simulink library "LowFrequencyNoiseEstimatorCoh"  (R2022b)
settings: Solver=VariableStepAuto  StartTime=0.0  StopTime=10.0  RelTol=1e-3
undefined symbols (not defined in the file or in its folder): decRate, magnitude, Row
libraries: TuneVar x22, StateVar x18, TOP x7, TSP x5, FeaturePath x3, HandyTextFile x2, matrix_library x2, PooliirLib x2, SpeedBoundsNoiseSlew x2, RfftLib x1, TunableDelay x1
settings Model: Creator=zs14328  LastModifiedBy=sc48041
settings SolverCC: AlgebraicLoopSolver=TrustRegion
settings DataIOCC: ReturnWorkspaceOutputs=off
settings DebuggingCC: UnconnectedInputMsg=warning  UnconnectedOutputMsg=warning  UnconnectedLineMsg=warning  SFMachineParentedDataDiag=warning  ArithmeticOperatorsInVariantConditions=warning
settings ModelReferenceCC: EnableRefExpFcnMdlSchedulingChecks=on
settings SFSimCC: CustomCodeUndefinedFunction=UseInterfaceOnly

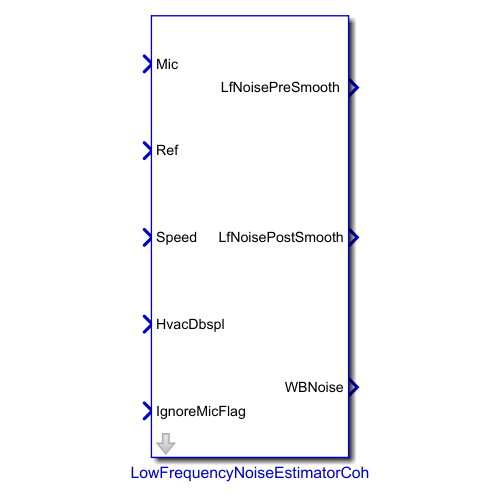
[thumbnail: Simulink's stored preview of the top-level diagram]
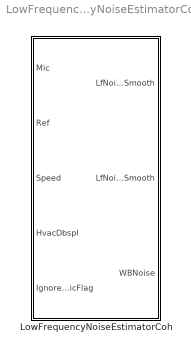
== system LowFrequencyNoiseEstimatorCoh ==
  LowFrequencyNoiseEstimatorCoh : Subsystem  mask(AudioPilot - Low-Frequency Noise Estimator){FeatureName=LfNoise, Config=[], TriggerInit=0}
      mask prompts: FeatureName "Feature Name:"; Config "LowFrequencyNoiseEstimatorCohConfig"
      mask help: This block implements the low-frequency noise estimator using the multi-coherence method.
      mask init:
      | blkh = gcbh;
      | 
      | Config = BTConfig.Assert(blkh,Config);
      | Config.Validate();
      | 
      | DecRate = Config.DecRateHz;
      | DecRate2 = Config.CoherenceDecRateHz;
      | DecRate3 = Config.CoherenceDecRate2Hz;
      | 
      | LowFrequencyNoiseEstimatorCohMask.ConfigureModel ...
      |                 (blkh,Config)
      | 
      | BTConfig.InitSetFeatureIfPresent(blkh,'FeatureName');
      mask Help:
      | This block implements the low-frequency noise estimator using the multi-coherence method.
      | 
      | Arguments for this block:
      | 
      | Design Time Configuration
      | The Feature Name can be specified unless a BTC instance is used, in which case, the instance name will be used as Feature Name.
      | 
      | Build Time Configuration
      | The block can be configured using a BTC object, LowFrequencyNoiseEstimatorCohConfig.
      mask TypeOptions FeatureName: FeaturePath/FeatureName
      mask Callback Config: BTConfig.CallbackHideIfPresent(gcbh,{'FeatureName'});
      mask Callback TriggerInit: LowFrequencyNoiseEstimatorCohMask.TriggerInitCallBack(gcbh);
      mask DialogControl DTCTitle Prompt: <b> Design Time Configuration </b>
      mask DialogControl BTCTitle Prompt: <b> Build Time Configuration </b>
      mask DialogControl Config Tooltip: The configuration has to be an object of the class, LowFrequencyNoiseEstimatorCohConfig.

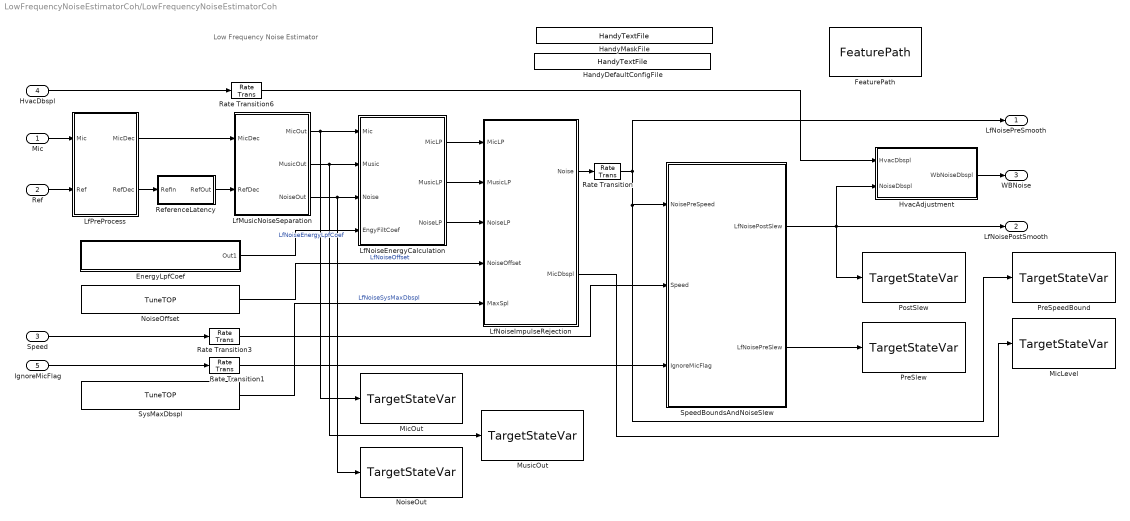
== system LowFrequencyNoiseEstimatorCoh/LowFrequencyNoiseEstimatorCoh ==
  note: Low Frequency Noise Estimator
  Mic : Inport
  Ref : Inport  Port=2
  Speed : Inport  Port=3
  HvacDbspl : Inport  Port=4
  IgnoreMicFlag : Inport  Port=5
  EnergyLpfCoef : Subsystem
  FeaturePath : FeaturePath/FeaturePath  FeatureName=LfNoise  IsGroup=off  GroupNumber=-1  IsModule=off  TriggerInit=[975 -106 1100 -39]
      settings: SourceProductName=Bose Talaria
  HandyDefaultConfigFile : HandyTextFile/HandyTextFile  TemplateSource=Config  FileSuffix=Init  OpenDialogOnLoad=off  UseThisBlockName=off  AddGrandParentNamePrefix=off  TheDefaultText=|  ShowInLibBrowser=on
      | % $(FILENAME) Setup model parameters for each "Init" callback (e.g. update diagram)
      | sample_rate_in_hertz = 44100;
      | frame_size = 32;
      | sysin_channel_count = 2;
      settings: SourceProductName=Bose Talaria
  HandyMaskFile : HandyTextFile/HandyTextFile  TemplateSource=<dialog fields>  FileSuffix=Mask  OpenDialogOnLoad=off  UseThisBlockName=off  AddGrandParentNamePrefix=off  TheDefaultText=|  ShowInLibBrowser=on
      | % $(FILENAME) Setup model parameters for each "Init" callback (e.g. update diagram)
      | sample_rate_in_hertz = 44100;
      | frame_size = 32;
      | sysin_channel_count = 2;
      settings: SourceProductName=Bose Talaria
  HvacAdjustment : Subsystem
  LfMusicNoiseSeparation : Subsystem
  LfNoiseEnergyCalculation : MATLAB Function  TreatAsAtomicUnit=on
  LfNoiseImpulseRejection : Subsystem
  LfPreProcess : Subsystem
  MicLevel : StateVar/TargetStateVar  TriggerInit=[1225 291 1365 359]  TspName=MicLevel  StateName=MicLevel  UseSameName=on  IfdefMacro=[]
      settings: SourceProductName=Bose Talaria
  MicOut : StateVar/TargetStateVar  TriggerInit=[335 366 475 434]  TspName=MicOut  StateName=MicOut  UseSameName=on  IfdefMacro=[]
      settings: SourceProductName=Bose Talaria
  MusicOut : StateVar/TargetStateVar  TriggerInit=[500 416 640 484]  TspName=MusicOut  StateName=MusicOut  UseSameName=on  IfdefMacro=[]
      settings: SourceProductName=Bose Talaria
  NoiseOffset : TuneVar/TuneTOP  TriggerInit=[-45 246 170 284]  TopName=OffsetDb  TuneName=OffsetDb  DataTypeOut=single  TunabilityNumber=1  MinValue=[]  MaxValue=[]  BankNumber=0  PreOverlay=false  PostOverlay=false  UseSameName=on  MaskValue=Config.NoiseOffsetDbspl
      settings: SourceProductName=Bose Talaria
  NoiseOut : StateVar/TargetStateVar  TriggerInit=[335 466 475 534]  TspName=NoiseOut  StateName=NoiseOut  UseSameName=on  IfdefMacro=[]
      settings: SourceProductName=Bose Talaria
  PostSlew : StateVar/TargetStateVar  TriggerInit=[1020 201 1160 269]  TspName=PostSlew  StateName=PostSlew  UseSameName=on  IfdefMacro=[]
      settings: SourceProductName=Bose Talaria
  PreSlew : StateVar/TargetStateVar  TriggerInit=[1020 296 1160 364]  TspName=PreSlew  StateName=PreSlew  UseSameName=on  IfdefMacro=[]
      settings: SourceProductName=Bose Talaria
  PreSpeedBound : StateVar/TargetStateVar  TriggerInit=[1225 201 1365 269]  TspName=PreSpeedBound  StateName=PreSpeedBound  UseSameName=on  IfdefMacro=[]
      settings: SourceProductName=Bose Talaria
  Rate Transition : RateTransition  OutPortSampleTime=1/DecRate2
  Rate Transition1 : RateTransition  Deterministic=off  OutPortSampleTime=1/DecRate2
  Rate Transition3 : RateTransition  Deterministic=off  OutPortSampleTime=1/DecRate2
  Rate Transition6 : RateTransition  Deterministic=off  OutPortSampleTimeOpt=Inherit  OutPortSampleTime=1/decRate
  ReferenceLatency : Subsystem
  SpeedBoundsAndNoiseSlew : Subsystem
  SysMaxDbspl : TuneVar/TuneTOP  TriggerInit=[-45 376 170 414]  TopName=SysMaxDbspl  TuneName=SysMaxDbspl  DataTypeOut=single  TunabilityNumber=1  MinValue=[]  MaxValue=[]  BankNumber=0  PreOverlay=false  PostOverlay=false  UseSameName=on  MaskValue=Config.SysMaxDbspl
      settings: SourceProductName=Bose Talaria
  "LfNoisePreSmooth " : Outport  VectorParamsAs1DForOutWhenUnconnected=off
  LfNoisePostSmooth : Outport  Port=2  VectorParamsAs1DForOutWhenUnconnected=off
  WBNoise : Outport  Port=3  VectorParamsAs1DForOutWhenUnconnected=off
  wires:
  Mic/1 -> LfPreProcess/1(Mic)
  Speed/1 -> Rate Transition3/1
  Ref/1 -> LfPreProcess/2(Ref)
  HvacAdjustment/1(WbNoiseDbspl) -> WBNoise/1
  HvacDbspl/1 -> Rate Transition6/1
  LfNoiseImpulseRejection/1(Noise) -> Rate Transition/1
  LfMusicNoiseSeparation/3(NoiseOut) -> NoiseOut/1, LfNoiseEnergyCalculation/3(Noise)
  LfMusicNoiseSeparation/1(MicOut) -> MicOut/1, LfNoiseEnergyCalculation/1(Mic)
  LfMusicNoiseSeparation/2(MusicOut) -> MusicOut/1, LfNoiseEnergyCalculation/2(Music)
  SpeedBoundsAndNoiseSlew/1(LfNoisePostSlew) -> PostSlew/1, LfNoisePostSmooth/1, HvacAdjustment/2(NoiseDbspl)
  LfNoiseImpulseRejection/2(MicDbspl) -> MicLevel/1
  SpeedBoundsAndNoiseSlew/2(LfNoisePreSlew) -> PreSlew/1
  EnergyLpfCoef/1(Out1) -> LfNoiseEnergyCalculation/4(EngyFiltCoef)  "LfNoiseEnergyLpfCoef"
  LfNoiseEnergyCalculation/1(MicLP) -> LfNoiseImpulseRejection/1(MicLP)
  LfNoiseEnergyCalculation/2(MusicLP) -> LfNoiseImpulseRejection/2(MusicLP)
  LfNoiseEnergyCalculation/3(NoiseLP) -> LfNoiseImpulseRejection/3(NoiseLP)
  NoiseOffset/1 -> LfNoiseImpulseRejection/4(NoiseOffset)  "LfNoiseOffset"
  LfPreProcess/2(RefDec) -> ReferenceLatency/1(RefIn)
  LfPreProcess/1(MicDec) -> LfMusicNoiseSeparation/1(MicDec)
  ReferenceLatency/1(RefOut) -> LfMusicNoiseSeparation/2(RefDec)
  Rate Transition3/1 -> SpeedBoundsAndNoiseSlew/2(Speed)
  Rate Transition6/1 -> HvacAdjustment/1(HvacDbspl)
  Rate Transition/1 -> "LfNoisePreSmooth "/1, PreSpeedBound/1, SpeedBoundsAndNoiseSlew/1(NoisePreSpeed)
  IgnoreMicFlag/1 -> Rate Transition1/1
  SysMaxDbspl/1 -> LfNoiseImpulseRejection/5(MaxSpl)  "LfNoiseSysMaxDbspl"
  Rate Transition1/1 -> SpeedBoundsAndNoiseSlew/3(IgnoreMicFlag)

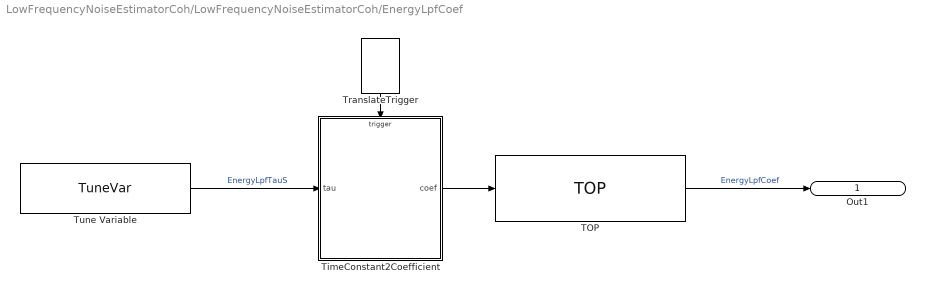
== system LowFrequencyNoiseEstimatorCoh/LowFrequencyNoiseEstimatorCoh/EnergyLpfCoef ==
  TOP : TOP/TOP  TriggerInit=[440 17 630 83]  TopName=EnergyLpfCoef  DataType=single  BankNumber=0  PreOverlay=false  PostOverlay=false  Role=Automatic
      settings: SourceProductName=Bose Talaria
  TimeConstant2Coefficient : MATLAB Function  TreatAsAtomicUnit=on
  TranslateTrigger : TuneVar/TranslateTrigger  TriggerInit=[306 -100 344 -45]
      settings: SourceProductName=Bose Talaria
  Tune Variable : TuneVar/TuneVar  TuneName=EnergyLpfTauS  SpecifyMaxSize=off  VariableDim=1 (Row)  MaxSize=[1 1]  TunabilityNumber=1  MinValue=[]  MaxValue=[]  TriggerInit=[-35 25 135 75]  MaskValue=Config.ImpRejEnergyFilterTauSec
      settings: SourceProductName=Bose Talaria
  Out1 : Outport  VectorParamsAs1DForOutWhenUnconnected=off
  wires:
  TOP/1 -> Out1/1  "EnergyLpfCoef"
  Tune Variable/1 -> TimeConstant2Coefficient/1(tau)  "EnergyLpfTauS"
  TimeConstant2Coefficient/1(coef) -> TOP/1
  TranslateTrigger/1 -> TimeConstant2Coefficient/Trigger

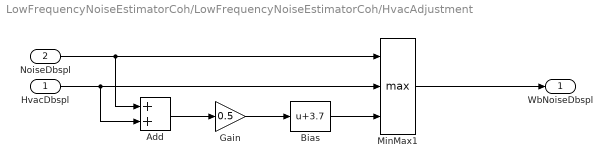
== system LowFrequencyNoiseEstimatorCoh/LowFrequencyNoiseEstimatorCoh/HvacAdjustment ==
  HvacDbspl : Inport
  NoiseDbspl : Inport  Port=2
  Add : Sum
  Bias : Bias  Bias=3.7  SaturateOnIntegerOverflow=off
  Gain : Gain  Gain=0.5
  MinMax1 : MinMax  Function=max  Inputs=3
  WbNoiseDbspl : Outport  VectorParamsAs1DForOutWhenUnconnected=off
  wires:
  NoiseDbspl/1 -> MinMax1/1, Add/1
  HvacDbspl/1 -> MinMax1/2, Add/2
  MinMax1/1 -> WbNoiseDbspl/1
  Add/1 -> Gain/1
  Gain/1 -> Bias/1
  Bias/1 -> MinMax1/3

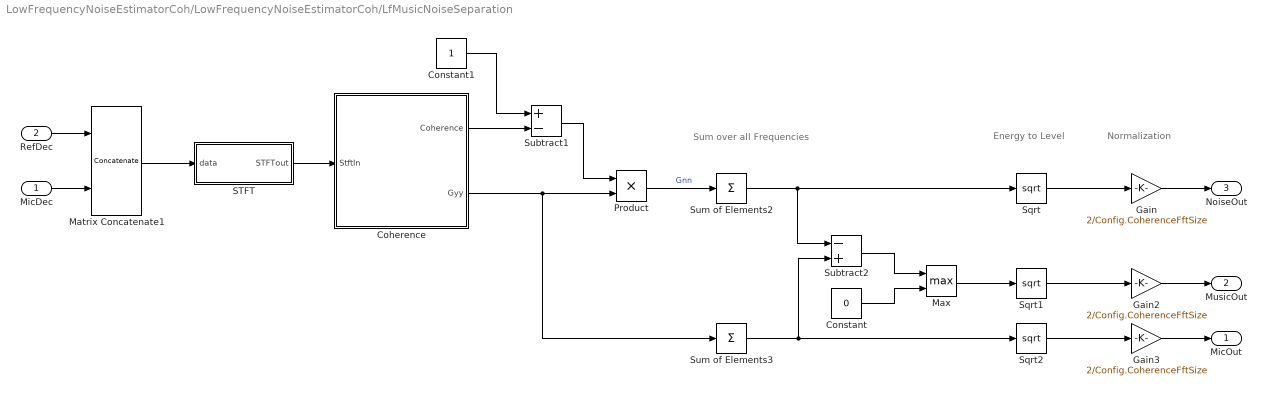
== system LowFrequencyNoiseEstimatorCoh/LowFrequencyNoiseEstimatorCoh/LfMusicNoiseSeparation ==
  note: Energy to
      | Level
  note: Sum over all
      | Frequencies
  note: Normalization
  MicDec : Inport
  RefDec : Inport  Port=2
  Coherence : Subsystem
  Constant : Constant  Value=0  OutDataTypeStr=single
  Constant1 : Constant  OutDataTypeStr=single
  Gain : Gain  Gain=2/Config.CoherenceFftSize
  Gain2 : Gain  Gain=2/Config.CoherenceFftSize
  Gain3 : Gain  Gain=2/Config.CoherenceFftSize
  Matrix Concatenate1 : Concatenate  Mode=Multidimensional array  ConcatenateDimension=2
  Max : MinMax  Function=max  Inputs=2
  Product : Product  RndMeth=Zero
  STFT : Subsystem
  Sqrt : Sqrt
  Sqrt1 : Sqrt
  Sqrt2 : Sqrt
  Subtract1 : Sum  Inputs=+-
  Subtract2 : Sum  Inputs=-+
  Sum of Elements2 : Sum  Inputs=+
  Sum of Elements3 : Sum  Inputs=+
  MicOut : Outport  VectorParamsAs1DForOutWhenUnconnected=off
  MusicOut : Outport  Port=2  VectorParamsAs1DForOutWhenUnconnected=off
  NoiseOut : Outport  Port=3  VectorParamsAs1DForOutWhenUnconnected=off
  wires:
  Coherence/1(Coherence) -> Subtract1/2
  Subtract1/1 -> Product/1
  Product/1 -> Sum of Elements2/1  "Gnn"
  Sum of Elements2/1 -> Subtract2/1, Sqrt/1
  Sqrt/1 -> Gain/1
  RefDec/1 -> Matrix Concatenate1/1
  MicDec/1 -> Matrix Concatenate1/2
  Constant1/1 -> Subtract1/1
  Coherence/2(Gyy) -> Product/2, Sum of Elements3/1
  Sum of Elements3/1 -> Sqrt2/1, Subtract2/2
  Sqrt2/1 -> Gain3/1
  Subtract2/1 -> Max/1
  Sqrt1/1 -> Gain2/1
  Gain/1 -> NoiseOut/1
  Gain2/1 -> MusicOut/1
  Gain3/1 -> MicOut/1
  Matrix Concatenate1/1 -> STFT/1(data)
  STFT/1(STFTout) -> Coherence/1(StftIn)
  Max/1 -> Sqrt1/1
  Constant/1 -> Max/2

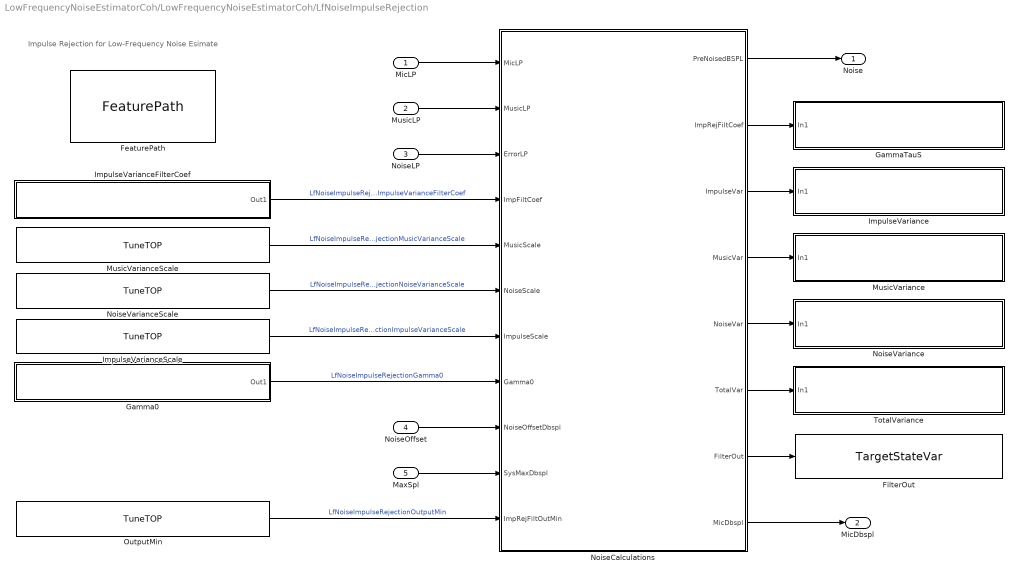
== system LowFrequencyNoiseEstimatorCoh/LowFrequencyNoiseEstimatorCoh/LfNoiseImpulseRejection ==
  note: Impulse Rejection for Low-Frequency Noise Esimate
  MicLP : Inport  SampleTime=1/DecRate3
  MusicLP : Inport  Port=2  SampleTime=1/DecRate3
  NoiseLP : Inport  Port=3  SampleTime=1/DecRate3
  NoiseOffset : Inport  Port=4
  MaxSpl : Inport  Port=5
  FeaturePath : FeaturePath/FeaturePath  FeatureName=ImpulseRejection  IsGroup=off  GroupNumber=-1  IsModule=off  TriggerInit=[-70 349 105 436]
      settings: SourceProductName=Bose Talaria
  FilterOut : StateVar/TargetStateVar  TriggerInit=[805 788 1055 842]  TspName=FilterOut  StateName=FilterOut  UseSameName=on  IfdefMacro=[]
      settings: SourceProductName=Bose Talaria
  Gamma0 : Subsystem
  GammaTauS : Subsystem
  ImpulseVariance : Subsystem
  ImpulseVarianceFilterCoef : Subsystem
  ImpulseVarianceScale : TuneVar/TuneTOP  TriggerInit=[-135 649 170 691]  TopName=ImpulseVarianceScale  TuneName=ImpulseVarianceScale  DataType=single  TunabilityNumber=1  MinValue=[]  MaxValue=[]  BankNumber=0  PreOverlay=false  PostOverlay=false  UseSameName=on  MaskValue=Config.ImpRejImpulseScale
      settings: SourceProductName=Bose Talaria
  MusicVariance : Subsystem
  MusicVarianceScale : TuneVar/TuneTOP  TriggerInit=[-135 539 170 581]  TopName=MusicVarianceScale  TuneName=MusicVarianceScale  DataType=single  TunabilityNumber=1  MinValue=[]  MaxValue=[]  BankNumber=0  PreOverlay=false  PostOverlay=false  UseSameName=on  MaskValue=Config.ImpRejMusicScale
      settings: SourceProductName=Bose Talaria
  NoiseCalculations : MATLAB Function  TreatAsAtomicUnit=on
  NoiseVariance : Subsystem
  NoiseVarianceScale : TuneVar/TuneTOP  TriggerInit=[-135 594 170 636]  TopName=NoiseVarianceScale  TuneName=NoiseVarianceScale  DataType=single  TunabilityNumber=1  MinValue=[]  MaxValue=[]  BankNumber=0  PreOverlay=false  PostOverlay=false  UseSameName=on  MaskValue=Config.ImpRejNoiseScale
      settings: SourceProductName=Bose Talaria
  "OutputMin " : TuneVar/TuneTOP  TriggerInit=[-135 869 170 911]  TopName=OutputMin  TuneName=OutputMin  DataType=single  TunabilityNumber=1  MinValue=[]  MaxValue=[]  BankNumber=0  PreOverlay=false  PostOverlay=false  UseSameName=on  MaskValue=Config.ImpRejOutputMin
      settings: SourceProductName=Bose Talaria
  TotalVariance : Subsystem
  Noise : Outport  VectorParamsAs1DForOutWhenUnconnected=off
  MicDbspl : Outport  Port=2  VectorParamsAs1DForOutWhenUnconnected=off
  wires:
  MicLP/1 -> NoiseCalculations/1(MicLP)
  MusicLP/1 -> NoiseCalculations/2(MusicLP)
  NoiseLP/1 -> NoiseCalculations/3(ErrorLP)
  "OutputMin "/1 -> NoiseCalculations/11(ImpRejFiltOutMin)  "LfNoiseImpulseRejectionOutputMin"
  NoiseCalculations/1(PreNoisedBSPL) -> Noise/1
  NoiseCalculations/8(MicDbspl) -> MicDbspl/1
  NoiseVarianceScale/1 -> NoiseCalculations/6(NoiseScale)  "LfNoiseImpulseRejectionNoiseVarianceScale"
  MusicVarianceScale/1 -> NoiseCalculations/5(MusicScale)  "LfNoiseImpulseRejectionMusicVarianceScale"
  ImpulseVarianceScale/1 -> NoiseCalculations/7(ImpulseScale)  "LfNoiseImpulseRejectionImpulseVarianceScale"
  Gamma0/1(Out1) -> NoiseCalculations/8(Gamma0)  "LfNoiseImpulseRejectionGamma0"
  ImpulseVarianceFilterCoef/1(Out1) -> NoiseCalculations/4(ImpFiltCoef)  "LfNoiseImpulseRejectionImpulseVarianceFilterCoef"
  MaxSpl/1 -> NoiseCalculations/10(SysMaxDbspl)
  NoiseOffset/1 -> NoiseCalculations/9(NoiseOffsetDbspl)
  NoiseCalculations/4(MusicVar) -> MusicVariance/1(In1)
  NoiseCalculations/3(ImpulseVar) -> ImpulseVariance/1(In1)
  NoiseCalculations/5(NoiseVar) -> NoiseVariance/1(In1)
  NoiseCalculations/6(TotalVar) -> TotalVariance/1(In1)
  NoiseCalculations/2(ImpRejFiltCoef) -> GammaTauS/1(In1)
  NoiseCalculations/7(FilterOut) -> FilterOut/1

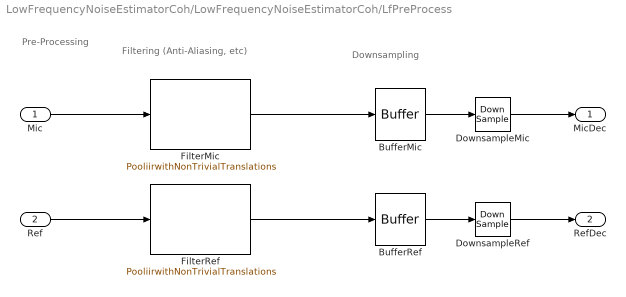
== system LowFrequencyNoiseEstimatorCoh/LowFrequencyNoiseEstimatorCoh/LfPreProcess ==
  note: Filtering
      | (Anti-Aliasing, etc)
  note: Downsampling
  note: Pre-Processing
  Mic : Inport
  Ref : Inport  Port=2
  BufferMic : Buffer  N=Config.DecimationFactor  OutputFrames=off
  BufferRef : Buffer  N=Config.DecimationFactor  OutputFrames=off
  DownsampleMic : DownSample  N=Config.DecimationFactor
  DownsampleRef : DownSample  N=Config.DecimationFactor
  FilterMic : PooliirLib/PooliirwithNonTrivialTranslations  maxNumStages=Config.AntiAliasFilterNumStages  numStages=Config.AntiAliasFilterNumStages  sosCoefficients=Config.AntiAliasFilterSos  alias='LPMicFilt'  variantType=Config.MicFiltVariant  FeatureName=Mic
  FilterRef : PooliirLib/PooliirwithNonTrivialTranslations  maxNumStages=Config.AntiAliasFilterNumStages  numStages=Config.AntiAliasFilterNumStages  sosCoefficients=Config.AntiAliasFilterSos  alias='LFRefFilt'  variantType=Config.RefFiltVariant  FeatureName=Ref
  MicDec : Outport  VectorParamsAs1DForOutWhenUnconnected=off
  RefDec : Outport  Port=2  VectorParamsAs1DForOutWhenUnconnected=off
  wires:
  DownsampleRef/1 -> RefDec/1
  DownsampleMic/1 -> MicDec/1
  BufferMic/1 -> DownsampleMic/1
  Mic/1 -> FilterMic/1
  Ref/1 -> FilterRef/1
  FilterMic/1 -> BufferMic/1
  BufferRef/1 -> DownsampleRef/1
  FilterRef/1 -> BufferRef/1

== system LowFrequencyNoiseEstimatorCoh/LowFrequencyNoiseEstimatorCoh/ReferenceLatency ==
  RefIn : Inport  SampleTime=1/DecRate
  Delay : TunableDelay/Delay  maxDelayTime=int32(floor(Config.RefMaxLatencyMsec/1000*DecRate))  frameSize=1  numChannels=1  bufferAlias=[]  headerFilename=[]
  RefLatencySamples : Subsystem
  RefOut : Outport  VectorParamsAs1DForOutWhenUnconnected=off
  wires:
  Delay/1 -> RefOut/1
  RefIn/1 -> Delay/1
  RefLatencySamples/1(LfNoiseRefLatencySamples) -> Delay/2  "LfNoise_ref_latency_samples"

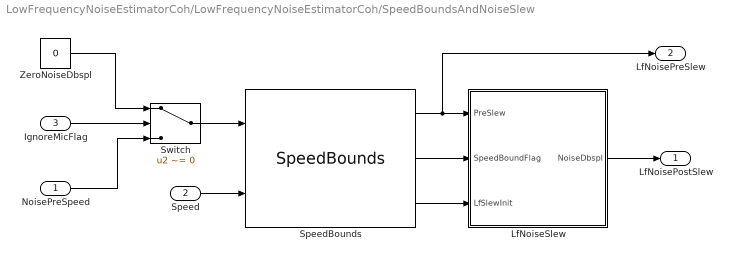
== system LowFrequencyNoiseEstimatorCoh/LowFrequencyNoiseEstimatorCoh/SpeedBoundsAndNoiseSlew ==
  NoisePreSpeed : Inport
  Speed : Inport  Port=2
  IgnoreMicFlag : Inport  Port=3
  LfNoiseSlew : Subsystem
  SpeedBounds : SpeedBoundsNoiseSlew/SpeedBounds  FeatureName=SpeedBounds  Config=Config.SpeedBounds
  Switch : Switch  Criteria=u2 ~= 0  SaturateOnIntegerOverflow=off  InputSameDT=off
  ZeroNoiseDbspl : Constant  Value=0  OutDataTypeStr=single
  LfNoisePostSlew : Outport  VectorParamsAs1DForOutWhenUnconnected=off
  LfNoisePreSlew : Outport  Port=2  VectorParamsAs1DForOutWhenUnconnected=off
  wires:
  Speed/1 -> SpeedBounds/2
  SpeedBounds/2 -> LfNoiseSlew/2(SpeedBoundFlag)
  SpeedBounds/1 -> LfNoisePreSlew/1, LfNoiseSlew/1(PreSlew)
  LfNoiseSlew/1(NoiseDbspl) -> LfNoisePostSlew/1
  NoisePreSpeed/1 -> Switch/3
  Switch/1 -> SpeedBounds/1
  IgnoreMicFlag/1 -> Switch/2
  ZeroNoiseDbspl/1 -> Switch/1
  SpeedBounds/3 -> LfNoiseSlew/3(LfSlewInit)

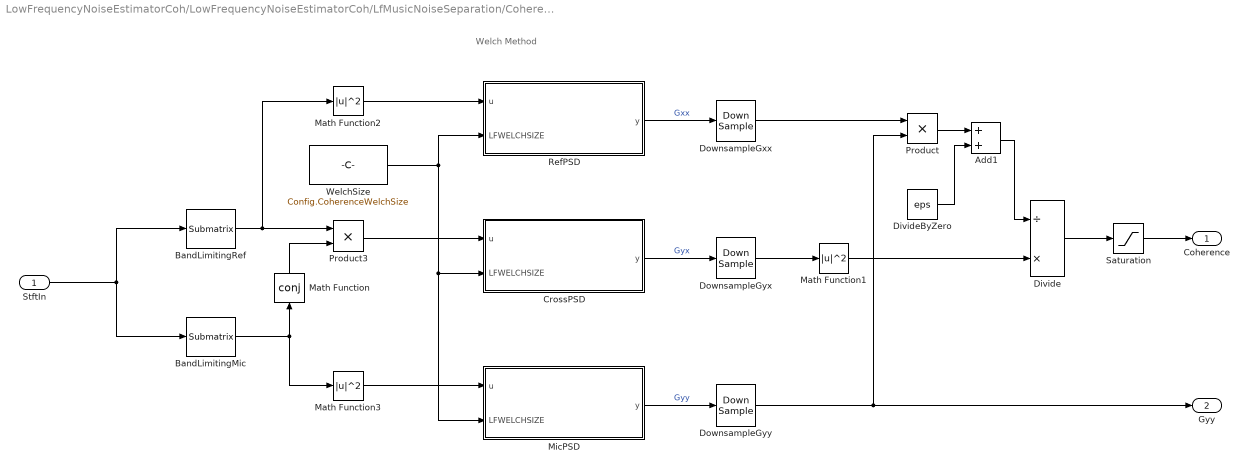
== system LowFrequencyNoiseEstimatorCoh/LowFrequencyNoiseEstimatorCoh/LfMusicNoiseSeparation/Coherence ==
  note: Welch Method
  StftIn : Inport
  Add1 : Sum
  BandLimitingMic : matrix_library/Submatrix  RowSpan=Range of rows  RowStartMode=Index  RowStartIndex=Config.CoherenceLowFrequencyIndex  RowEndMode=Index  RowEndIndex=Config.CoherenceHighFrequencyIndex  ColSpan=One column  ColStartMode=Last  ColStartIndex=1  ColEndMode=Last  ColEndIndex=1
  BandLimitingRef : matrix_library/Submatrix  RowSpan=Range of rows  RowStartMode=Index  RowStartIndex=Config.CoherenceLowFrequencyIndex  RowEndMode=Index  RowEndIndex=Config.CoherenceHighFrequencyIndex  ColSpan=One column  ColStartMode=First  ColStartIndex=1  ColEndMode=Index  ColEndIndex=1
  CrossPSD : MATLAB Function  TreatAsAtomicUnit=on
  Divide : Product  Inputs=/*
  DivideByZero : Constant  Value=eps  OutDataTypeStr=single
  DownsampleGxx : DownSample  N=Config.CoherenceWelchSize  RateOptions=Allow multirate processing
  DownsampleGyx : DownSample  N=Config.CoherenceWelchSize  RateOptions=Allow multirate processing
  DownsampleGyy : DownSample  N=Config.CoherenceWelchSize  RateOptions=Allow multirate processing
  Math Function : Math  Operator=conj  SignedPower=on
  Math Function1 : Math  Operator=magnitude^2  SignedPower=on
  Math Function2 : Math  Operator=magnitude^2  SignedPower=on
  Math Function3 : Math  Operator=magnitude^2  SignedPower=on
  MicPSD : MATLAB Function  TreatAsAtomicUnit=on
  Product : Product  RndMeth=Zero
  Product3 : Product  RndMeth=Zero
  "RefPSD " : MATLAB Function  TreatAsAtomicUnit=on
  Saturation : Saturate  UpperLimit=1  LowerLimit=0
  WelchSize : Constant  Value=Config.CoherenceWelchSize  OutDataTypeStr=single
  Coherence : Outport  VectorParamsAs1DForOutWhenUnconnected=off
  Gyy : Outport  Port=2  VectorParamsAs1DForOutWhenUnconnected=off
  wires:
  Math Function/1 -> Product3/2
  Divide/1 -> Saturation/1
  Product3/1 -> CrossPSD/1(u)
  StftIn/1 -> BandLimitingMic/1, BandLimitingRef/1
  Product/1 -> Add1/1
  Math Function1/1 -> Divide/2
  CrossPSD/1(y) -> DownsampleGyx/1  "Gyx"
  "RefPSD "/1(y) -> DownsampleGxx/1  "Gxx"
  MicPSD/1(y) -> DownsampleGyy/1  "Gyy"
  DivideByZero/1 -> Add1/2
  Add1/1 -> Divide/1
  Math Function2/1 -> "RefPSD "/1(u)
  Math Function3/1 -> MicPSD/1(u)
  BandLimitingRef/1 -> Product3/1, Math Function2/1
  BandLimitingMic/1 -> Math Function/1, Math Function3/1
  WelchSize/1 -> "RefPSD "/2(LFWELCHSIZE), MicPSD/2(LFWELCHSIZE), CrossPSD/2(LFWELCHSIZE)
  DownsampleGxx/1 -> Product/1
  DownsampleGyx/1 -> Math Function1/1
  DownsampleGyy/1 -> Product/2, Gyy/1
  Saturation/1 -> Coherence/1

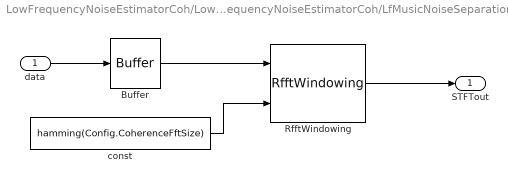
== system LowFrequencyNoiseEstimatorCoh/LowFrequencyNoiseEstimatorCoh/LfMusicNoiseSeparation/STFT ==
  data : Inport
  Buffer : Buffer  N=Config.CoherenceFftSize  V=Config.CoherenceOverlap
  RfftWindowing : RfftLib/RfftWindowing  Description=This block computes the Fourier Transform using an optimized FFT for real 2-channel input.  Config=Config.RfftWindowingStft
      settings: SourceProductName=Bose Blocklib
  const : Constant  Value=hamming(Config.CoherenceFftSize)  OutDataTypeStr=single
  STFTout : Outport  VectorParamsAs1DForOutWhenUnconnected=off
  wires:
  Buffer/1 -> RfftWindowing/1
  const/1 -> RfftWindowing/2
  data/1 -> Buffer/1
  RfftWindowing/1 -> STFTout/1

== system LowFrequencyNoiseEstimatorCoh/LowFrequencyNoiseEstimatorCoh/LfNoiseImpulseRejection/Gamma0 ==
  TOP : TOP/TOP  TriggerInit=[475 20 675 70]  TopName=Gamma0  DataType=single  BankNumber=0  PreOverlay=false  PostOverlay=false  Role=Automatic
      settings: SourceProductName=Bose Talaria
  TimeConstant2Coefficient : MATLAB Function  TreatAsAtomicUnit=on
  TranslateTrigger : TuneVar/TranslateTrigger  TriggerInit=[306 -100 344 -45]
      settings: SourceProductName=Bose Talaria
  Tune Variable : TuneVar/TuneVar  TuneName=Gamma0TauS  SpecifyMaxSize=off  VariableDim=1 (Row)  MaxSize=[1 1]  TunabilityNumber=1  MinValue=[]  MaxValue=[]  TriggerInit=[-160 22 155 68]  MaskValue=Config.ImpRejGamma0TauSec
      settings: SourceProductName=Bose Talaria
  Out1 : Outport  VectorParamsAs1DForOutWhenUnconnected=off
  wires:
  TOP/1 -> Out1/1  "Gamma0"
  Tune Variable/1 -> TimeConstant2Coefficient/1(tau)  "Gamma0TauS"
  TimeConstant2Coefficient/1(coef) -> TOP/1
  TranslateTrigger/1 -> TimeConstant2Coefficient/Trigger

== system LowFrequencyNoiseEstimatorCoh/LowFrequencyNoiseEstimatorCoh/LfNoiseImpulseRejection/GammaTauS ==
  In1 : Inport
  GammaConversion : MATLAB Function  TreatAsAtomicUnit=on
  InterpretTrigger : StateVar/InterpretTrigger  TriggerInit=[336 20 374 75]
      settings: SourceProductName=Bose Talaria
  StateVar : StateVar/StateVar  TriggerInit=[495 139 735 201]  StateName=GammaTauS
      settings: SourceProductName=Bose Talaria
  TSP : TSP/TSP  TriggerInit=[0 138 260 202]  TspName=FiltCoef  IfDefMacro=[]  Role=Automatic
      settings: SourceProductName=Bose Talaria
  wires:
  InterpretTrigger/1 -> GammaConversion/Trigger
  TSP/1 -> GammaConversion/1(Coef)
  GammaConversion/1(State) -> StateVar/1
  In1/1 -> TSP/1

== system LowFrequencyNoiseEstimatorCoh/LowFrequencyNoiseEstimatorCoh/LfNoiseImpulseRejection/ImpulseVariance ==
  In1 : Inport
  InterpretTrigger : StateVar/InterpretTrigger  TriggerInit=[336 20 374 75]
      settings: SourceProductName=Bose Talaria
  StateVar : StateVar/StateVar  TriggerInit=[495 139 735 201]  StateName=ImpulseVarianceDb
      settings: SourceProductName=Bose Talaria
  TSP : TSP/TSP  TriggerInit=[0 138 215 202]  TspName=ImpulseVariance  IfDefMacro=[]  Role=Automatic
      settings: SourceProductName=Bose Talaria
  db20 : MATLAB Function  TreatAsAtomicUnit=on
  wires:
  In1/1 -> TSP/1
  db20/1(State) -> StateVar/1
  TSP/1 -> db20/1(TSP1)
  InterpretTrigger/1 -> db20/Trigger

== system LowFrequencyNoiseEstimatorCoh/LowFrequencyNoiseEstimatorCoh/LfNoiseImpulseRejection/ImpulseVarianceFilterCoef ==
  TOP : TOP/TOP  TriggerInit=[440 17 725 83]  TopName=ImpulseVarianceFilterCoef  DataType=single  BankNumber=0  PreOverlay=false  PostOverlay=false  Role=Automatic
      settings: SourceProductName=Bose Talaria
  TimeConstant2Coefficient : MATLAB Function  TreatAsAtomicUnit=on
  TranslateTrigger : TuneVar/TranslateTrigger  TriggerInit=[306 -100 344 -45]
      settings: SourceProductName=Bose Talaria
  Tune Variable : TuneVar/TuneVar  TuneName=ImpulseVarianceFiltTauS  SpecifyMaxSize=off  VariableDim=1 (Row)  MaxSize=[1 1]  TunabilityNumber=1  MinValue=[]  MaxValue=[]  TriggerInit=[-265 20 100 80]  MaskValue=Config.ImpRejImpulseVarianceFilterTauSec
      settings: SourceProductName=Bose Talaria
  Out1 : Outport  VectorParamsAs1DForOutWhenUnconnected=off
  wires:
  TOP/1 -> Out1/1  "ImpulseVarianceFilterCoef"
  Tune Variable/1 -> TimeConstant2Coefficient/1(tau)  "ImpulseVarianceFiltTauS"
  TimeConstant2Coefficient/1(coef) -> TOP/1
  TranslateTrigger/1 -> TimeConstant2Coefficient/Trigger

== system LowFrequencyNoiseEstimatorCoh/LowFrequencyNoiseEstimatorCoh/LfNoiseImpulseRejection/MusicVariance ==
  In1 : Inport
  InterpretTrigger : StateVar/InterpretTrigger  TriggerInit=[336 20 374 75]
      settings: SourceProductName=Bose Talaria
  StateVar : StateVar/StateVar  TriggerInit=[455 136 685 204]  StateName=MusicVarianceDb
      settings: SourceProductName=Bose Talaria
  TSP : TSP/TSP  TriggerInit=[20 136 260 204]  TspName=MusicVariance  IfDefMacro=[]  Role=Automatic
      settings: SourceProductName=Bose Talaria
  "db20 " : MATLAB Function  TreatAsAtomicUnit=on
  wires:
  In1/1 -> TSP/1
  "db20 "/1(State) -> StateVar/1
  TSP/1 -> "db20 "/1(TSP1)
  InterpretTrigger/1 -> "db20 "/Trigger

== system LowFrequencyNoiseEstimatorCoh/LowFrequencyNoiseEstimatorCoh/LfNoiseImpulseRejection/NoiseVariance ==
  In1 : Inport
  InterpretTrigger : StateVar/InterpretTrigger  TriggerInit=[336 20 374 75]
      settings: SourceProductName=Bose Talaria
  StateVar : StateVar/StateVar  TriggerInit=[455 136 685 204]  StateName=NoiseVarianceDb
      settings: SourceProductName=Bose Talaria
  TSP : TSP/TSP  TriggerInit=[20 136 260 204]  TspName=NoiseVariance  IfDefMacro=[]  Role=Automatic
      settings: SourceProductName=Bose Talaria
  "db20 " : MATLAB Function  TreatAsAtomicUnit=on
  wires:
  InterpretTrigger/1 -> "db20 "/Trigger
  TSP/1 -> "db20 "/1(TSP1)
  "db20 "/1(State) -> StateVar/1
  In1/1 -> TSP/1

== system LowFrequencyNoiseEstimatorCoh/LowFrequencyNoiseEstimatorCoh/LfNoiseImpulseRejection/TotalVariance ==
  In1 : Inport
  InterpretTrigger : StateVar/InterpretTrigger  TriggerInit=[336 20 374 75]
      settings: SourceProductName=Bose Talaria
  StateVar : StateVar/StateVar  TriggerInit=[455 136 685 204]  StateName=TotalVarianceDb
      settings: SourceProductName=Bose Talaria
  TSP : TSP/TSP  TriggerInit=[20 136 260 204]  TspName=TotalVariance  IfDefMacro=[]  Role=Automatic
      settings: SourceProductName=Bose Talaria
  "db20 " : MATLAB Function  TreatAsAtomicUnit=on
  wires:
  InterpretTrigger/1 -> "db20 "/Trigger
  TSP/1 -> "db20 "/1(TSP1)
  "db20 "/1(State) -> StateVar/1
  In1/1 -> TSP/1

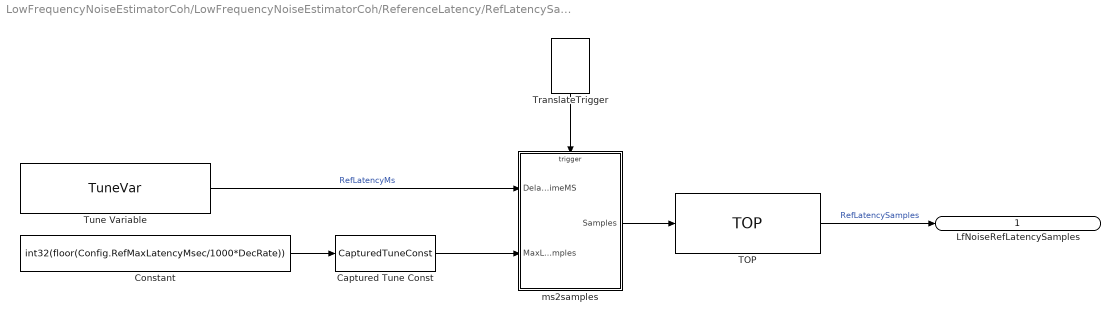
== system LowFrequencyNoiseEstimatorCoh/LowFrequencyNoiseEstimatorCoh/ReferenceLatency/RefLatencySamples ==
  Captured Tune Const : TuneVar/CapturedTuneConst  TriggerInit=[70 162 170 198]  Role=Automatic
      settings: SourceProductName=Bose Talaria
  Constant : Constant  Value=int32(floor(Config.RefMaxLatencyMsec/1000*DecRate))  OutDataTypeStr=int32
  TOP : TOP/TOP  TriggerInit=[410 120 555 180]  TopName=RefLatencySamples  DataType=int32  BankNumber=0  PreOverlay=false  PostOverlay=false  Role=Automatic
      settings: SourceProductName=Bose Talaria
  TranslateTrigger : TuneVar/TranslateTrigger  TriggerInit=[286 -35 324 20]
      settings: SourceProductName=Bose Talaria
  Tune Variable : TuneVar/TuneVar  TuneName=RefLatencyMs  SpecifyMaxSize=off  VariableDim=1 (Row)  MaxSize=[1 1]  TunabilityNumber=1  MinValue=[]  MaxValue=[]  TriggerInit=[-245 90 -55 140]  MaskValue=Config.RefLatencyMsec
      settings: SourceProductName=Bose Talaria
  ms2samples : MATLAB Function  TreatAsAtomicUnit=on
  LfNoiseRefLatencySamples : Outport  VectorParamsAs1DForOutWhenUnconnected=off
  wires:
  Tune Variable/1 -> ms2samples/1(DelayTimeMS)  "RefLatencyMs"
  ms2samples/1(Samples) -> TOP/1
  TranslateTrigger/1 -> ms2samples/Trigger
  TOP/1 -> LfNoiseRefLatencySamples/1  "RefLatencySamples"
  Captured Tune Const/1 -> ms2samples/2(MaxLatencySamples)
  Constant/1 -> Captured Tune Const/1

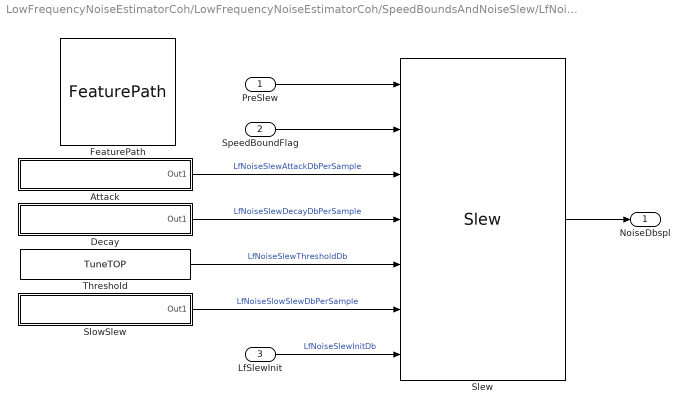
== system LowFrequencyNoiseEstimatorCoh/LowFrequencyNoiseEstimatorCoh/SpeedBoundsAndNoiseSlew/LfNoiseSlew ==
  PreSlew : Inport
  SpeedBoundFlag : Inport  Port=2
  LfSlewInit : Inport  Port=3
  Attack : Subsystem
  Decay : Subsystem
  FeaturePath : FeaturePath/FeaturePath  FeatureName=Slew  IsGroup=off  GroupNumber=-1  IsModule=off  TriggerInit=[-225 44 -110 151]
      settings: SourceProductName=Bose Talaria
  Slew : SpeedBoundsNoiseSlew/Slew  SystemSampleTime=-1  VariantActivationTime=update diagram  Latency=0  AutoFrameSizeCalculation=off
  SlowSlew : Subsystem
  Threshold : TuneVar/TuneTOP  TriggerInit=[-265 255 -95 285]  TopName=ThresholdDb  TuneName=ThresholdDb  DataType=single  TunabilityNumber=1  MinValue=[]  MaxValue=[]  BankNumber=0  PreOverlay=false  PostOverlay=false  UseSameName=on  MaskValue=Config.SlewThresholdDb
      settings: SourceProductName=Bose Talaria
  NoiseDbspl : Outport  VectorParamsAs1DForOutWhenUnconnected=off
  wires:
  Slew/1 -> NoiseDbspl/1
  SpeedBoundFlag/1 -> Slew/2
  PreSlew/1 -> Slew/1
  SlowSlew/1(Out1) -> Slew/6  "LfNoiseSlowSlewDbPerSample"
  Attack/1(Out1) -> Slew/3  "LfNoiseSlewAttackDbPerSample"
  Threshold/1 -> Slew/5  "LfNoiseSlewThresholdDb"
  Decay/1(Out1) -> Slew/4  "LfNoiseSlewDecayDbPerSample"
  LfSlewInit/1 -> Slew/7  "LfNoiseSlewInitDb"

== system LowFrequencyNoiseEstimatorCoh/LowFrequencyNoiseEstimatorCoh/SpeedBoundsAndNoiseSlew/LfNoiseSlew/Attack ==
  TOP : TOP/TOP  TriggerInit=[125 85 330 145]  TopName=AttackDbPerSample  DataType=single  BankNumber=0  PreOverlay=false  PostOverlay=false  Role=Automatic
      settings: SourceProductName=Bose Talaria
  TranslateTrigger : TuneVar/TranslateTrigger  TriggerInit=[-19 -10 19 45]
      settings: SourceProductName=Bose Talaria
  Tune Variable : TuneVar/TuneVar  TuneName=AttackDbPerS  SpecifyMaxSize=off  VariableDim=1 (Row)  MaxSize=[1 1]  TunabilityNumber=1  MinValue=[]  MaxValue=[]  TriggerInit=[-385 90 -215 140]  MaskValue=Config.SlewAttackDbpersec
      settings: SourceProductName=Bose Talaria
  sec2sample : MATLAB Function  TreatAsAtomicUnit=on
  Out1 : Outport  VectorParamsAs1DForOutWhenUnconnected=off
  wires:
  TOP/1 -> Out1/1  "AttackDbPerSample"
  sec2sample/1(y) -> TOP/1
  Tune Variable/1 -> sec2sample/1(u)  "AttackDbPerS"
  TranslateTrigger/1 -> sec2sample/Trigger

== system LowFrequencyNoiseEstimatorCoh/LowFrequencyNoiseEstimatorCoh/SpeedBoundsAndNoiseSlew/LfNoiseSlew/Decay ==
  TOP : TOP/TOP  TriggerInit=[100 85 315 145]  TopName=DecayDbPerSample  DataType=single  BankNumber=0  PreOverlay=false  PostOverlay=false  Role=Automatic
      settings: SourceProductName=Bose Talaria
  TranslateTrigger : TuneVar/TranslateTrigger  TriggerInit=[-19 -10 19 45]
      settings: SourceProductName=Bose Talaria
  Tune Variable : TuneVar/TuneVar  TuneName=DecayDbPerS  SpecifyMaxSize=off  VariableDim=1 (Row)  MaxSize=[1 1]  TunabilityNumber=1  MinValue=[]  MaxValue=[]  TriggerInit=[-385 90 -215 140]  MaskValue=Config.SlewDecayDbpersec
      settings: SourceProductName=Bose Talaria
  sec2sample : MATLAB Function  TreatAsAtomicUnit=on
  Out1 : Outport  VectorParamsAs1DForOutWhenUnconnected=off
  wires:
  TranslateTrigger/1 -> sec2sample/Trigger
  Tune Variable/1 -> sec2sample/1(u)  "DecayDbPerS"
  sec2sample/1(y) -> TOP/1
  TOP/1 -> Out1/1  "DecayDbPerSample"

== system LowFrequencyNoiseEstimatorCoh/LowFrequencyNoiseEstimatorCoh/SpeedBoundsAndNoiseSlew/LfNoiseSlew/SlowSlew ==
  TOP : TOP/TOP  TriggerInit=[100 87 320 143]  TopName=SlowDbPerSample  DataType=single  BankNumber=0  PreOverlay=false  PostOverlay=false  Role=Automatic
      settings: SourceProductName=Bose Talaria
  TranslateTrigger : TuneVar/TranslateTrigger  TriggerInit=[-19 -10 19 45]
      settings: SourceProductName=Bose Talaria
  Tune Variable : TuneVar/TuneVar  TuneName=SlowDbPerS  SpecifyMaxSize=off  VariableDim=1 (Row)  MaxSize=[1 1]  TunabilityNumber=1  MinValue=[]  MaxValue=[]  TriggerInit=[-335 90 -165 140]  MaskValue=Config.SlewSlowSlewDbpersec
      settings: SourceProductName=Bose Talaria
  sec2sample : MATLAB Function  TreatAsAtomicUnit=on
  Out1 : Outport  VectorParamsAs1DForOutWhenUnconnected=off
  wires:
  TOP/1 -> Out1/1  "SlowDbPerSample"
  sec2sample/1(y) -> TOP/1
  Tune Variable/1 -> sec2sample/1(u)  "SlowDbPerS"
  TranslateTrigger/1 -> sec2sample/Trigger

== matlab function LowFrequencyNoiseEstimatorCoh/LfNoiseImpulseRejection/MusicVariance/db20  ==
  data: State output; TSP1 input
  events: trigger input FUNCTION_CALL_EVENT
function State  = fcn(TSP1)
%#codegen

State = db20(abs(TSP1) + eps);

== matlab function LowFrequencyNoiseEstimatorCoh/SpeedBoundsAndNoiseSlew/LfNoiseSlew/SlowSlew/sec2sample ==
  data: u input; y output; DecRate2 parameter
  events: trigger input FUNCTION_CALL_EVENT
function y = fcn(u, DecRate2)
% Convert rate from per second to per sample

y = u.Value/DecRate2;

== matlab function LowFrequencyNoiseEstimatorCoh/LfNoiseImpulseRejection/ImpulseVarianceFilterCoef/TimeConstant2Coefficient ==
  data: coef output; tau input; DecRate3 parameter
  events: trigger input FUNCTION_CALL_EVENT
function coef  = fcn(tau,DecRate3)
% Convert time constant to filter coefficient
%#codegen

wc = 1/(DecRate3*tau.Value);
coef = (1-sin(wc))/cos(wc);

== matlab function LowFrequencyNoiseEstimatorCoh/LfNoiseImpulseRejection/Gamma0/TimeConstant2Coefficient ==
  data: coef output; tau input; DecRate3 parameter
  events: trigger input FUNCTION_CALL_EVENT
function coef  = fcn(tau,DecRate3)
% Convert time constant to filter coefficient
%#codegen

wc = 1/(DecRate3*tau.Value);
coef = (1-sin(wc))/cos(wc);

== matlab function LowFrequencyNoiseEstimatorCoh/EnergyLpfCoef/TimeConstant2Coefficient ==
  data: coef output; tau input; DecRate3 parameter
  events: trigger input FUNCTION_CALL_EVENT
function coef  = fcn(tau,DecRate3)
% Convert time constant to filter coefficient
%#codegen

wc = 1/(DecRate3*tau.Value);
coef = (1-sin(wc))/cos(wc);

== matlab function LowFrequencyNoiseEstimatorCoh/LfNoiseEnergyCalculation ==
  data: Mic input; MicLP output; Music input; Noise input; EngyFiltCoef input; MusicLP output; NoiseLP output
function [MicLP, MusicLP, NoiseLP] ...
  = EnergyCalc(Mic, Music, Noise, EngyFiltCoef)
% Energy salculation has been simplified from before
% This is now just a smoothing of the output from the
% coherence calculations.

% States 
persistent MusicLPState NoiseLPState MicLPState;

% Initialization
if isempty(MusicLPState) 
    MusicLPState = single(0);	
end
if isempty(NoiseLPState)
    NoiseLPState = single(0);
end
if isempty(MicLPState)
    MicLPState = single(0);
end

% Energy Conversion
MusicLPState     = MusicLPState*EngyFiltCoef ...
	+ abs(Music)*(1-EngyFiltCoef);
NoiseLPState     = NoiseLPState*EngyFiltCoef ...
	+ abs(Noise)*(1-EngyFiltCoef);
MicLPState       = MicLPState*EngyFiltCoef ...
	+ abs(Mic)*(1-EngyFiltCoef);

% Output
MusicLP = MusicLPState;
NoiseLP = NoiseLPState;
MicLP = MicLPState;

== matlab function LowFrequencyNoiseEstimatorCoh/LfNoiseImpulseRejection/ImpulseVariance/db20 ==
  data: State output; TSP1 input
  events: trigger input FUNCTION_CALL_EVENT
function State  = fcn(TSP1)
%#codegen

State = db20(abs(TSP1)+eps);

== matlab function LowFrequencyNoiseEstimatorCoh/LfNoiseImpulseRejection/NoiseVariance/db20  ==
  data: State output; TSP1 input
  events: trigger input FUNCTION_CALL_EVENT
function State  = fcn(TSP1)
%#codegen

State = db20(abs(TSP1) + eps);

== matlab function LowFrequencyNoiseEstimatorCoh/LfNoiseImpulseRejection/TotalVariance/db20  ==
  data: State output; TSP1 input
  events: trigger input FUNCTION_CALL_EVENT
function State  = fcn(TSP1)
%#codegen

State = db20(abs(TSP1) + eps);

== matlab function LowFrequencyNoiseEstimatorCoh/LfNoiseImpulseRejection/GammaTauS/GammaConversion ==
  data: State output; Coef input; DecRate3 parameter
  events: trigger input FUNCTION_CALL_EVENT
function State  = fcn(Coef,DecRate3)
% Converts the filter coefficient back to time constant
%#codegen

% Keep all values single
one1 = single(1.0);
zero1 = single(0.0);

% Handle the divide-by-zero case
if (Coef == one1)
    State = zero1;
else
    State = one1 / ((one1 - Coef)*DecRate3);
end

== matlab function LowFrequencyNoiseEstimatorCoh/ReferenceLatency/RefLatencySamples/ms2samples ==
  data: DelayTimeMS input; MaxLatencySamples input; Samples output; DecRate parameter
  events: trigger input FUNCTION_CALL_EVENT
function Samples = fcn(DelayTimeMS, MaxLatencySamples, DecRate)
% Convert from milliseconds to samples

% Use floor to minimize the risk of going noncausal 
Samples = floor(DelayTimeMS.Value*DecRate/1000);


if Samples > MaxLatencySamples
    TranslateError('Delay amount cannot be greater than specified max delay');
end

== matlab function LowFrequencyNoiseEstimatorCoh/LfMusicNoiseSeparation/Coherence/RefPSD  ==
  data: u input; y output; LFWELCHSIZE input
function y = fcn(u,LFWELCHSIZE)
% This function forms the power spectral density over
% LFWELCHSIZE frames.

K = LFWELCHSIZE;

%#eml
% Double States
persistent counter;
persistent Psd;             % Holds the PSD accumulation
persistent prevout;         % Contains the previous PSD
if isempty(counter) counter = 0; end
if isempty(Psd)     Psd = single(zeros(size(u))); end
if isempty(prevout) prevout = single(zeros(size(u))); end

% Increment the counter
counter = counter + 1;

% The output is the previous PSD for K frames until
% the next PSD is ready
if counter < K
    Psd = Psd + u/K;
    y = prevout;
elseif counter ==K
    y = Psd;
    prevout = Psd;
    Psd = single(zeros(size(u)));
    counter = 0;
else
    y = prevout;
end

end

== matlab function LowFrequencyNoiseEstimatorCoh/LfMusicNoiseSeparation/Coherence/CrossPSD ==
  data: u input; y output; LFWELCHSIZE input
function y = fcn(u,LFWELCHSIZE)
% This function forms the power spectral density over
% LFWELCHSIZE frames.

K = LFWELCHSIZE;

%#eml
% Double States
persistent counter;
persistent Psd;             % Holds the PSD accumulation
persistent prevout;         % Contains the previous PSD
if isempty(counter) counter = 0; end
if isempty(Psd)     Psd = complex(single(zeros(size(u)))); end
if isempty(prevout) prevout = complex(single(zeros(size(u)))); end

% Increment the counter
counter = counter + 1;

% The output is the previous PSD for K frames until
% the next PSD is ready
if counter < K
    Psd = Psd + u/K;
    y = prevout;
elseif counter ==K
    y = Psd;
    prevout = Psd;
    Psd = complex(single(zeros(size(u))));
    counter = 0;
else
    y = prevout;
end

end

== matlab function LowFrequencyNoiseEstimatorCoh/LfMusicNoiseSeparation/Coherence/MicPSD ==
  data: u input; y output; LFWELCHSIZE input
function y = fcn(u,LFWELCHSIZE)
% This function forms the power spectral density over
% LFWELCHSIZE frames.

K = LFWELCHSIZE;

%#eml
% Double States
persistent counter;
persistent Psd;             % Holds the PSD accumulation
persistent prevout;         % Contains the previous PSD
if isempty(counter) counter = 0; end
if isempty(Psd)     Psd = single(zeros(size(u))); end
if isempty(prevout) prevout = single(zeros(size(u))); end

% Increment the counter
counter = counter + 1;

% The output is the previous PSD for K frames until
% the next PSD is ready
if counter < K
    Psd = Psd + u/K;
    y = prevout;
elseif counter ==K
    y = Psd;
    prevout = Psd;
    Psd = single(zeros(size(u)));
    counter = 0;
else
    y = prevout;
end

end

== matlab function LowFrequencyNoiseEstimatorCoh/SpeedBoundsAndNoiseSlew/LfNoiseSlew/Attack/sec2sample ==
  data: u input; y output; DecRate2 parameter
  events: trigger input FUNCTION_CALL_EVENT
function y = fcn(u, DecRate2)
% Convert rate from per second to per sample

y = u.Value/DecRate2;

== matlab function LowFrequencyNoiseEstimatorCoh/LfNoiseImpulseRejection/NoiseCalculations ==
  data: MicLP input size=1; MusicLP input; ErrorLP input; ImpFiltCoef input =inflation; MusicScale input =musicScale; NoiseScale input =noiseScale; ImpulseScale input =impulseScale; Gamma0 input; NoiseOffsetDbspl input =noiseOffsetdBSPL; SysMaxDbspl input =sysMaxdBSPL; PreNoisedBSPL output single; ImpRejFiltCoef output; ImpulseVar output; MusicVar output; NoiseVar output; TotalVar output; FilterOut output; ImpRejFiltOutMin input; MicDbspl output
function [PreNoisedBSPL, ImpRejFiltCoef, ...
    ImpulseVar, MusicVar, NoiseVar, ...
    TotalVar, FilterOut, MicDbspl] ...
  = NoiseCalc(MicLP, MusicLP, ErrorLP, ...
        ImpFiltCoef,...
        MusicScale, NoiseScale, ImpulseScale,...
        Gamma0,...
        NoiseOffsetDbspl, SysMaxDbspl,...
        ImpRejFiltOutMin)
% Function that conditions the noise energy.
% Performs impulse rejection
% Microphone energy check
% Convert to dBSPL
% Also outputs various intermediate check points
   
% States
% Initialize to zero
persistent ImpFiltState FiltOut;
if isempty(ImpFiltState) 
    ImpFiltState = single([0 0]);
end
if isempty(FiltOut)
    FiltOut   = single(ImpRejFiltOutMin);
end

% Impulse Estimate
% A First-Order Filter is applied twice
ImpFiltState(1) = ImpFiltState(1)*ImpFiltCoef ...
	+ ErrorLP*(1-ImpFiltCoef);
ImpFiltState(2) = ImpFiltState(2)*ImpFiltCoef ...
	+ ImpFiltState(1)*(1-ImpFiltCoef);

% Variances & Scaling
MusicVar = MusicScale * MusicLP^2;
NoiseVar = NoiseScale * ImpFiltState(2)^2;
ImpulseVar = ImpulseScale ...
	* (max(0, ErrorLP-ImpFiltState(2)))^2;
TotalVar = NoiseVar + max(0, MusicVar+ImpulseVar);

% Gamma correction
ImpRejFiltCoef = 1 - Gamma0*NoiseVar/(TotalVar+eps);

% Impulse Reject Filter
FiltOut = ImpRejFiltCoef*FiltOut+ErrorLP*(1-ImpRejFiltCoef);

% Set Minimum Bound
FiltOut = max(FiltOut, ImpRejFiltOutMin);

% Filter Output
FilterOut = FiltOut;

% dBSPL Conversion and Microphone Energy Check
PreNoisedBSPL = db20(FiltOut+eps)...
	+ NoiseOffsetDbspl + SysMaxDbspl;

% Microphone Level
MicDbspl= db20(MicLP)+SysMaxDbspl+NoiseOffsetDbspl;

return
end

function y = db20(x)
y = 20*log10(abs(x));
return;
end

== matlab function LowFrequencyNoiseEstimatorCoh/SpeedBoundsAndNoiseSlew/LfNoiseSlew/Decay/sec2sample ==
  data: u input; y output; DecRate2 parameter
  events: trigger input FUNCTION_CALL_EVENT
function y = fcn(u, DecRate2)
% Convert rate from per second to per sample

y = -abs(u.Value/DecRate2);
